simulink model "PositionControlFuzzy"  (R2022b)
settings: Solver=FixedStepAuto  StartTime=0.0  StopTime=100.0  FixedStep=Ts  RelTol=1e-3
undefined symbols (not defined in the file): DiscIntNeverNeededParam, refx, refy
libraries: fuzblock x1
settings Model: Creator=pizarro  LastModifiedBy=lublu
settings SolverCC: AlgebraicLoopSolver=TrustRegion
settings DataIOCC: ReturnWorkspaceOutputs=off
settings OptimizationCC: ReuseModelBlockBuffer=on
settings DebuggingCC: UnconnectedInputMsg=warning  UnconnectedOutputMsg=warning  UnconnectedLineMsg=warning
settings ModelReferenceCC: EnableRefExpFcnMdlSchedulingChecks=on
settings SFSimCC: CustomCodeUndefinedFunction=UseInterfaceOnly

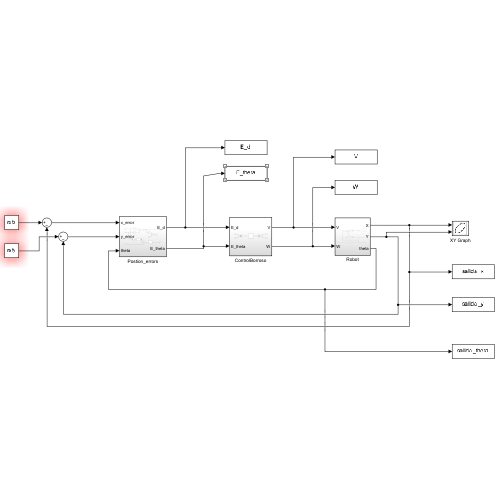
[thumbnail: Simulink's stored preview of the top-level diagram]
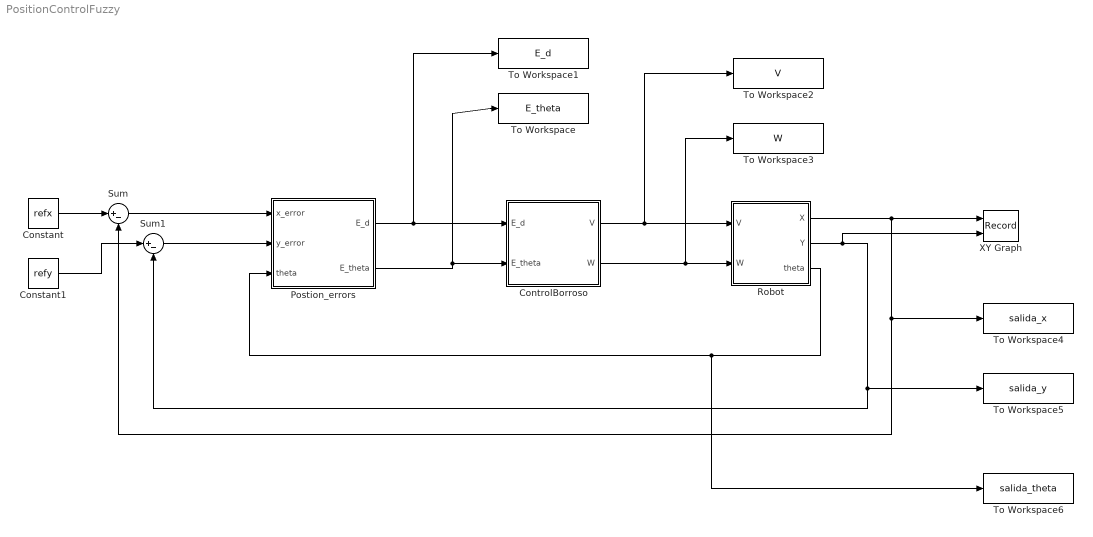
== system PositionControlFuzzy ==
  Constant : Constant  Value=refx
  Constant1 : Constant  Value=refy
  ControlBorroso : Subsystem
  Postion_errors : Subsystem
  Robot : Subsystem
  Sum : Sum  Inputs=|+-
  Sum1 : Sum  Inputs=|+-
  To Workspace : ToWorkspace  VariableName=E_theta  SaveFormat=Structure With Time  SampleTime=-1
  To Workspace1 : ToWorkspace  VariableName=E_d  SaveFormat=Structure With Time  SampleTime=-1
  To Workspace2 : ToWorkspace  VariableName=V  SaveFormat=Structure With Time  SampleTime=-1
  To Workspace3 : ToWorkspace  VariableName=W  SaveFormat=Structure With Time  SampleTime=-1
  To Workspace4 : ToWorkspace  VariableName=salida_x  SaveFormat=Structure With Time  SampleTime=-1
  To Workspace5 : ToWorkspace  VariableName=salida_y  SaveFormat=Structure With Time  SampleTime=-1
  To Workspace6 : ToWorkspace  VariableName=salida_theta  SaveFormat=Structure With Time  SampleTime=-1
  XY Graph : Record  FileSettingsInternal="{\"entries\":[{\"content\":{\"excelSettings\":{\"content\":{},\"type\":\"Streamout.ExcelSettings\"}},\"type\":\"Streamout.FileSettingStorage\",\"uuid\":\"\"}],\"packageUris\":[\"http:\\/\\/schema.mathworks.com\\/mf0\\/streamout_blocks\\/R2020a\"],\"version\":\"1.0\"}"  Layout=[1 1]  SignalsInternal="{\"entries\":[{\"content\":{\"signals\":[{\"content\":{\"blockPath\":[],\"channel\":[],\"dimensions\":[1],\"domain\":\"\",\"lineColor\":\"#a2142f\",\"plots\":[1],\"port\":1,\"sid\":[],\"signalID\":8,\"signalName\":\"Robot:1\"},\"type\":\"RecordBlkView.Signal\",\"uuid\":\"\"},{\"content\":{\"blockPath\":[],\"channel\":[],\"dimensions\":[1],\"domain\":\"\",\"lineColor\":\"#139fff\",\"plots\":[1],\"port\":2,\"sid\":[],\"signalID\":11,\"signalName\":\"Robot:2\"},\"type\":\"RecordBlkView.Signal\",\"uuid\":\"\"}]},\"type\":\"RecordBlkView.InputSignals\",\"uuid\":\"\"}],\"packageUris\":[\"http:\\/\\/schema.mathworks.com\\/mf0\\/streamout_blocks\\/R2020a\"],\"version\":\"1.0\"}"  VisualizationBindings="{\"xyplotplugin\":{\"info\":[{\"series\":[{\"bindingParametersList\":[{\"parameter\":\"X-Axis\",\"signalID\":8,\"signalName\":\"Robot:1\"},{\"parameter\":\"Y-Axis\",\"signalID\":11,\"signalName\":\"Robot:2\"}],\"seriesID\":41546}],\"subplotID\":1}]}}"  CompatibilityTag=XY
  wires:
  Postion_errors/1(E_d) -> ControlBorroso/1(E_d), To Workspace1/1
  Postion_errors/2(E_theta) -> ControlBorroso/2(E_theta), To Workspace/1
  Sum1/1 -> Postion_errors/2(y_error)
  Sum/1 -> Postion_errors/1(x_error)
  Constant/1 -> Sum/1
  Constant1/1 -> Sum1/1
  Robot/1(X) -> XY Graph/1, Sum/2, To Workspace4/1
  Robot/2(Y) -> XY Graph/2, Sum1/2, To Workspace5/1
  Robot/3(theta) -> To Workspace6/1, Postion_errors/3(theta)
  ControlBorroso/2(W) -> To Workspace3/1, Robot/2(W)
  ControlBorroso/1(V) -> To Workspace2/1, Robot/1(V)

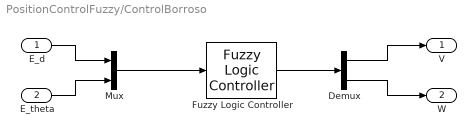
== system PositionControlFuzzy/ControlBorroso ==
  E_d : Inport
  E_theta : Inport  Port=2
  Demux : Demux  Outputs=2
  Fuzzy Logic Controller : fuzblock/Fuzzy Logic  Controller  FIS='ControlBorroso.fis'  OutputSampleNumber=101  DataType=double  FuzzifiedInputs=off  RuleFiringStrengths=off  RuleOutputs=off  AggregatedOutputs=off  SimulateUsing=Interpreted execution  OutOfRangeInputValueMessage=warning  NoRuleFiredMessage=warning  EmptyOutputFuzzySetMessage=warning
  Mux : Mux  Inputs=2
  V : Outport
  W : Outport  Port=2
  wires:
  E_theta/1 -> Mux/2
  E_d/1 -> Mux/1
  Mux/1 -> Fuzzy Logic Controller/1
  Fuzzy Logic Controller/1 -> Demux/1
  Demux/2 -> W/1
  Demux/1 -> V/1

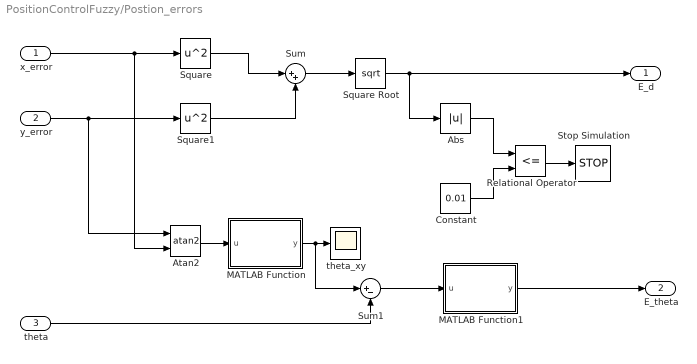
== system PositionControlFuzzy/Postion_errors ==
  x_error : Inport
  y_error : Inport  Port=2
  theta : Inport  Port=3
  Abs : Abs  SaturateOnIntegerOverflow=off
  Atan2 : Trigonometry  Operator=atan2
  Constant : Constant  Value=0.01
  MATLAB Function : MATLAB Function  TreatAsAtomicUnit=on
  MATLAB Function1 : MATLAB Function  TreatAsAtomicUnit=on
  Relational Operator : RelationalOperator  Operator=<=  OutDataTypeStr=boolean  RndMeth=Simplest  InputSameDT=off
  Square : Math  Operator=square
  Square Root : Sqrt
  Square1 : Math  Operator=square
  Stop Simulation : Stop
  Sum : Sum  Inputs=|++
  Sum1 : Sum  Inputs=|+-
  theta_xy : Scope
  E_d : Outport
  E_theta : Outport  Port=2
  wires:
  x_error/1 -> Atan2/2, Square/1
  Abs/1 -> Relational Operator/1
  MATLAB Function/1(y) -> Sum1/1, theta_xy/1
  Square Root/1 -> E_d/1, Abs/1
  Atan2/1 -> MATLAB Function/1(u)
  Sum/1 -> Square Root/1
  Sum1/1 -> MATLAB Function1/1(u)
  Constant/1 -> Relational Operator/2
  Relational Operator/1 -> Stop Simulation/1
  MATLAB Function1/1(y) -> E_theta/1
  Square1/1 -> Sum/2
  Square/1 -> Sum/1
  y_error/1 -> Atan2/1, Square1/1
  theta/1 -> Sum1/2

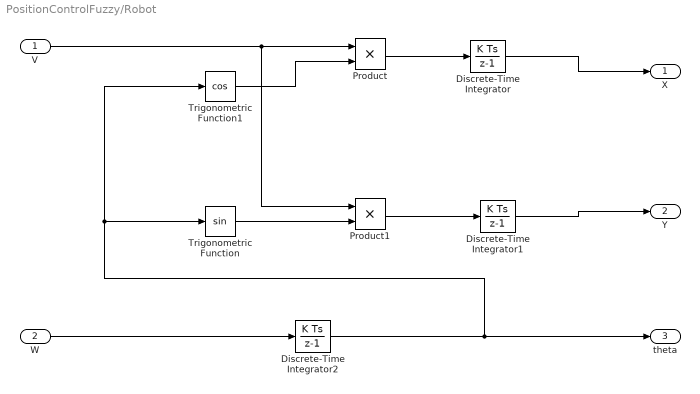
== system PositionControlFuzzy/Robot ==
  V : Inport
  W : Inport  Port=2
  Discrete-Time Integrator : DiscreteIntegrator  SampleTime=-1  ICPrevOutput=DiscIntNeverNeededParam  ICPrevScaledInput=DiscIntNeverNeededParam
  Discrete-Time Integrator1 : DiscreteIntegrator  SampleTime=-1  ICPrevOutput=DiscIntNeverNeededParam  ICPrevScaledInput=DiscIntNeverNeededParam
  Discrete-Time Integrator2 : DiscreteIntegrator  SampleTime=-1  ICPrevOutput=DiscIntNeverNeededParam  ICPrevScaledInput=DiscIntNeverNeededParam
  Product : Product
  Product1 : Product
  Trigonometric Function : Trigonometry
  Trigonometric Function1 : Trigonometry  Operator=cos
  X : Outport
  Y : Outport  Port=2
  theta : Outport  Port=3
  wires:
  Trigonometric Function1/1 -> Product/2
  Product1/1 -> Discrete-Time Integrator1/1
  Trigonometric Function/1 -> Product1/2
  Discrete-Time Integrator2/1 -> theta/1, Trigonometric Function1/1, Trigonometric Function/1
  Product/1 -> Discrete-Time Integrator/1
  Discrete-Time Integrator1/1 -> Y/1
  V/1 -> Product1/1, Product/1
  Discrete-Time Integrator/1 -> X/1
  W/1 -> Discrete-Time Integrator2/1

== matlab function PositionControlFuzzy/Postion_errors/MATLAB Function ==
  data: u input; y output
function y = fcn(u)
    if u<-pi
        u=u+2*pi;
    end
    if u>pi
        u=u-2*pi;
    end
y = u;

== matlab function PositionControlFuzzy/Postion_errors/MATLAB Function1 ==
  data: u input; y output
function y = fcn(u)
    if u<-pi
        u=u+2*pi;
    end
    if u>pi
        u=u-2*pi;
    end
y = u;
